simulink model "MassSDamper"  (R2021a)
settings: Solver=VariableStepAuto  StartTime=0.0  StopTime=10.0  MaxStep=1e-3  RelTol=1e-3
values from neighbouring files (symbols this model uses):
  b = 10    [MassSpringDamper.m]
  k = 400    [MassSpringDamper.m]
  m = massValues(i)    [MassSpringDamper.m]
  x0 = 1    [MassSpringDamper.m]
settings Model: Creator=lenovo  LastModifiedBy=lenovo

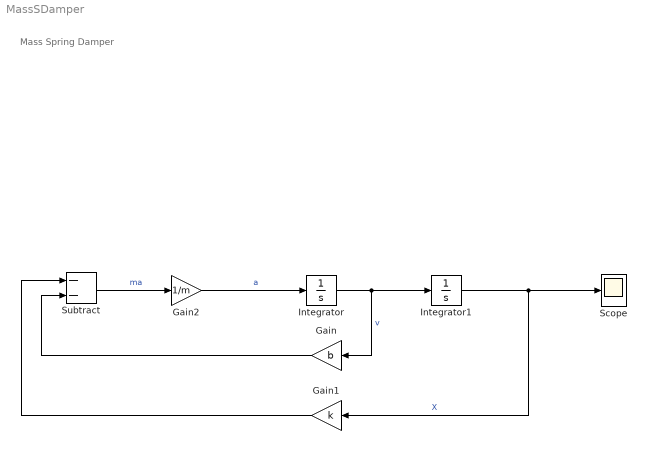
== system MassSDamper ==
  note: Mass Spring Damper
  Gain : Gain  Gain=b
  Gain1 : Gain  Gain=k
  Gain2 : Gain  Gain=1/m
  Integrator : Integrator
  Integrator1 : Integrator  InitialCondition=x0
  Scope : Scope
  Subtract : Sum  Inputs=--
  wires:
  Gain2/1 -> Integrator/1  "a"
  Integrator/1 -> Gain/1, Integrator1/1  "v"
  Integrator1/1 -> Scope/1, Gain1/1  "X"
  Gain/1 -> Subtract/2
  Gain1/1 -> Subtract/1
  Subtract/1 -> Gain2/1  "ma"
